simulink model "APB_Model0_v03_Test"  (R2020b)
settings: Solver=ode45  StartTime=0.0  StopTime=inf  RelTol=1e-3
undefined symbols (not defined in the file or in its folder): calb_Driver_acce, calb_Driver_bttn, calb_Driver_EmrBrk, calb_Driver_Prss, G_Fclamp, G_Kmot, G_Rmot, G_Stroke, G_SwOmega, GEN3, PbcDataStorageRequest_t
libraries: etargetslib x26, Lib_Op_Hndl x4, simulink x2, PbcOut_Checksum x2
(part 1 of 5)
settings Model: DataDictionary=APB_ModelDic.sldd  Creator=ISA1DRY  LastModifiedBy=OMO1DRY
settings SolverCC: ZeroCrossControl=DisableAll  ZeroCrossAlgorithm=Adaptive
settings DebuggingCC: IgnoredZcDiagnostic=none

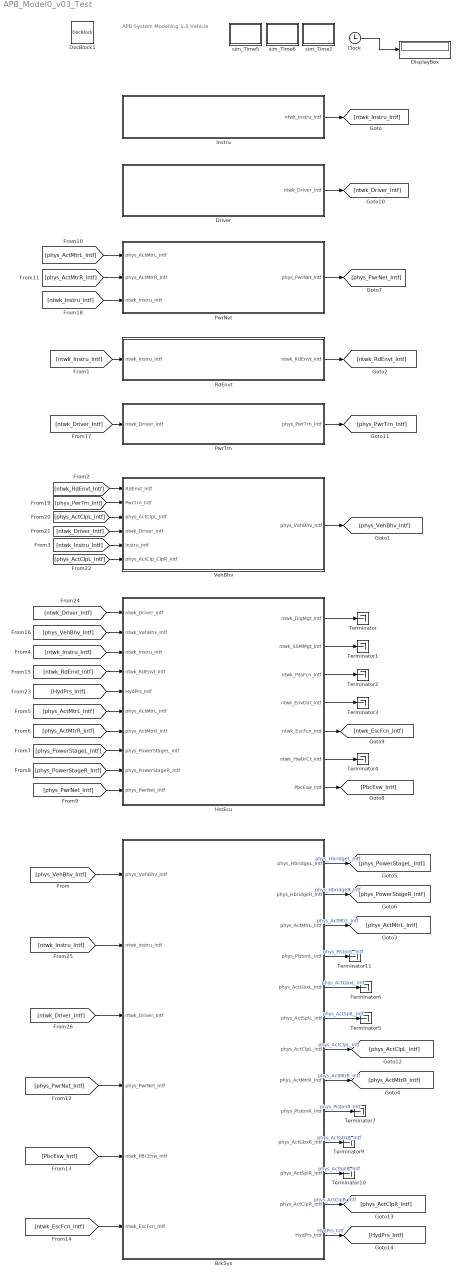
== system APB_Model0_v03_Test ==
  note: APB System Modelling
      | 1.0 Vehicle
  BrkSys : Subsystem
  Clock : Clock
  DisplayBox : Display
  DocBlock1 : simulink/Model-Wide Utilities/DocBlock  DocumentType=Text
      content=|
      | TyDate = 5 May 2023
      | Updated by = ALI ISSA
      | Model name = APB System Modeling
      | level = 02
      | version = 03
      |
      | Description
      |
      | New APB Model with the improved architecture...
  Driver : Subsystem
  HstEcu : Subsystem
  Instru : Subsystem
  PwrNet : Subsystem
  PwrTrn : Subsystem
  RdEnvt : Subsystem
  Terminator{,1..7,9..11} (11 alike) : Terminator
  VehBhv : Subsystem
  sim_Time1 : Subsystem
      mask Display: disp('Plot');
  sim_Time5 : Subsystem
      settings: OpenFcn=clear;
      mask Display: disp('clear');
  sim_Time6 : Subsystem
      settings: OpenFcn=|
      | startupNew_2;
      | Data_IntegDRYJPN3;
      mask Display: disp('load\nstartup');
  wires:
  Instru/1(ntwk_Instru_Intf) -> [ntwk_Instru_Intf]
  Driver/1(ntwk_Driver_Intf) -> [ntwk_Driver_Intf]
  [ntwk_Instru_Intf] -> RdEnvt/1(ntwk_Instru_Intf)
  [phys_ActMtrL_Intf] -> PwrNet/1(phys_ActMtrL_Intf)
  [phys_ActMtrR_Intf] -> PwrNet/2(phys_ActMtrR_Intf)
  [ntwk_Instru_Intf] -> PwrNet/3(ntwk_Instru_Intf)
  PwrNet/1(phys_PwrNet_Intf) -> [phys_PwrNet_Intf]
  RdEnvt/1(ntwk_RdEnvt_Intf) -> [ntwk_RdEnvt_Intf]
  [ntwk_Driver_Intf] -> PwrTrn/1(ntwk_Driver_Intf)
  PwrTrn/1(phys_PwrTrn_Intf) -> [phys_PwrTrn_Intf]
  [ntwk_RdEnvt_Intf] -> VehBhv/1(RdEnvt_Intf)
  VehBhv/1(phys_VehBhv_Intf) -> [phys_VehBhv_Intf]
  [phys_PwrTrn_Intf] -> VehBhv/2(PwrTrn_Intf)
  [phys_ActClpL_Intf] -> VehBhv/3(phys_ActClpL_Intf)
  [ntwk_Driver_Intf] -> VehBhv/4(ntwk_Driver_Intf)
  [ntwk_Instru_Intf] -> VehBhv/5(Instru_Intf)
  [phys_ActClpL_Intf] -> VehBhv/6(phys_ActClp_ClpR_Intf)
  [phys_PowerStageL_Intf] -> HstEcu/8(phys_PowerStageL_Intf)
  [phys_PowerStageR_Intf] -> HstEcu/9(phys_PowerStageR_Intf)
  [phys_PwrNet_Intf] -> HstEcu/10(phys_PwrNet_Intf)
  [phys_ActMtrL_Intf] -> HstEcu/6(phys_ActMtrL_Intf)
  [ntwk_Driver_Intf] -> HstEcu/1(ntwk_Driver_Intf)
  [phys_VehBhv_Intf] -> HstEcu/2(ntwk_VehBhv_Intf)
  [ntwk_Instru_Intf] -> HstEcu/3(ntwk_Instru_Intf)
  [ntwk_RdEnvt_Intf] -> HstEcu/4(ntwk_RdEnvt_Intf)
  [HydPrs_Intf] -> HstEcu/5(HydPrs_Intf)
  [phys_ActMtrR_Intf] -> HstEcu/7(phys_ActMtrR_Intf)
  HstEcu/7(PbcEsw_Intf) -> [PbcEsw_Intf]
  HstEcu/5(ntwk_EscFcn_Intf) -> [ntwk_EscFcn_Intf]
  HstEcu/1(ntwk_DigMgt_Intf) -> Terminator/1
  HstEcu/3(ntwk_PdsFcn_Intf) -> Terminator2/1
  HstEcu/2(ntwk_SSMMgt_Intf) -> Terminator1/1
  HstEcu/4(ntwk_EnvDat_Intf) -> Terminator3/1
  HstEcu/6(ntwk_HwDrCt_Intf) -> Terminator4/1
  [phys_PwrNet_Intf] -> BrkSys/4(phys_PwrNet_Intf)
  [PbcEsw_Intf] -> BrkSys/5(ntwk_PBCEsw_Intf)
  [ntwk_EscFcn_Intf] -> BrkSys/6(ntwk_EscFcn_Intf)
  [phys_VehBhv_Intf] -> BrkSys/1(phys_VehBhv_Intf)
  [ntwk_Instru_Intf] -> BrkSys/2(ntwk_Instru_Intf)
  [ntwk_Driver_Intf] -> BrkSys/3(ntwk_Driver_Intf)
  BrkSys/13(HydPrs_Intf) -> [HydPrs_Intf]  "HydPrs_Intf"
  BrkSys/1(phys_HbridgeL_Intf) -> [phys_PowerStageL_Intf]  "phys_HbridgeL_Intf"
  BrkSys/2(phys_HbridgeR_Intf) -> [phys_PowerStageR_Intf]  "phys_HbridgeR_Intf"
  BrkSys/3(phys_ActMtrL_Intf) -> [phys_ActMtrL_Intf]  "phys_ActMtrL_Intf"
  BrkSys/8(phys_ActMtrR_Intf) -> [phys_ActMtrR_Intf]  "phys_ActMtrR_Intf"
  BrkSys/5(phys_ActGbxL_Intf) -> Terminator6/1  "phys_ActGbxL_Intf"
  BrkSys/6(phys_ActSplL_Intf) -> Terminator5/1  "phys_ActSplL_Intf"
  BrkSys/7(phys_ActClpL_Intf) -> [phys_ActClpL_Intf]  "phys_ActClpL_Intf"
  BrkSys/11(phys_ActSplR_Intf) -> Terminator10/1  "phys_ActSplR_Intf"
  BrkSys/12(phys_ActClpR_Intf) -> [phys_ActClpR_Intf]  "phys_ActClpR_Intf"
  BrkSys/10(phys_ActGbxR_Intf) -> Terminator9/1  "phys_ActGbxR_Intf"
  BrkSys/4(phys_PistonL_Intf) -> Terminator11/1  "phys_PistonL_Intf"
  BrkSys/9(phys_PistonR_Intf) -> Terminator7/1  "phys_PistonR_Intf"
  Clock/1 -> DisplayBox/1

== system APB_Model0_v03_Test/BrkSys ==
  phys_VehBhv_Intf : Inport
  ntwk_Instru_Intf : Inport  Port=2
  ntwk_Driver_Intf : Inport  Port=3
  phys_PwrNet_Intf : Inport  Port=4
  ntwk_PBCEsw_Intf : Inport  Port=5
  ntwk_EscFcn_Intf : Inport  Port=6
  Subsystem Reference : Subsystem  ReferencedSubsystem=Ssys_BrkSysAPB_v02_0
  phys_HbridgeL_Intf : Outport
  phys_HbridgeR_Intf : Outport  Port=2
  phys_ActMtrL_Intf : Outport  Port=3
  phys_PistonL_Intf : Outport  Port=4
  phys_ActGbxL_Intf : Outport  Port=5
  phys_ActSplL_Intf : Outport  Port=6
  phys_ActClpL_Intf : Outport  Port=7
  phys_ActMtrR_Intf : Outport  Port=8
  phys_PistonR_Intf : Outport  Port=9
  phys_ActGbxR_Intf : Outport  Port=10
  phys_ActSplR_Intf : Outport  Port=11
  phys_ActClpR_Intf : Outport  Port=12
  HydPrs_Intf : Outport  Port=13
  wires:
  Subsystem Reference/9 -> phys_ActGbxR_Intf/1  "phys_ActGbxR_Intf"
  Subsystem Reference/4 -> phys_ActGbxL_Intf/1  "phys_ActGbxL_Intf"
  Subsystem Reference/12 -> phys_HbridgeR_Intf/1  "phys_HbridgeR_Intf"
  Subsystem Reference/13 -> HydPrs_Intf/1  "HydPrs_Intf"
  Subsystem Reference/8 -> phys_PistonR_Intf/1  "phys_PistonR_Intf"
  ntwk_EscFcn_Intf/1 -> Subsystem Reference/6
  Subsystem Reference/11 -> phys_ActClpR_Intf/1  "phys_ActClpR_Intf"
  Subsystem Reference/7 -> phys_ActMtrR_Intf/1  "phys_ActMtrR_Intf"
  Subsystem Reference/3 -> phys_PistonL_Intf/1  "phys_PistonL_Intf"
  Subsystem Reference/10 -> phys_ActSplR_Intf/1  "phys_ActSplR_Intf"
  phys_VehBhv_Intf/1 -> Subsystem Reference/1
  Subsystem Reference/6 -> phys_ActClpL_Intf/1  "phys_ActClpL_Intf"
  ntwk_Instru_Intf/1 -> Subsystem Reference/2
  ntwk_Driver_Intf/1 -> Subsystem Reference/3
  Subsystem Reference/5 -> phys_ActSplL_Intf/1  "phys_ActSplL_Intf"
  Subsystem Reference/1 -> phys_HbridgeL_Intf/1  "phys_HbridgeL_Intf"
  phys_PwrNet_Intf/1 -> Subsystem Reference/4
  ntwk_PBCEsw_Intf/1 -> Subsystem Reference/5
  Subsystem Reference/2 -> phys_ActMtrL_Intf/1  "phys_ActMtrL_Intf"

== system APB_Model0_v03_Test/Driver ==
  Cmpt_DriverAPB_v01_0_Test : Subsystem
  Subsystem1 : Subsystem
  ntwk_Driver_Intf : Outport
  wires:
  Cmpt_DriverAPB_v01_0_Test/1(calb_Driver_bttn) -> Subsystem1/1(calb_Driver_bttn)  "calb_Driver_bttn"
  Cmpt_DriverAPB_v01_0_Test/2(calb_Driver_Prss) -> Subsystem1/2(calb_Driver_Prss)  "calb_Driver_Prss"
  Cmpt_DriverAPB_v01_0_Test/4(calb_Driver_EmrBrk) -> Subsystem1/4(calb_Driver_EmrBrk)  "calb_Driver_EmrBrk"
  Subsystem1/1(ntwk_Driver_Intf) -> ntwk_Driver_Intf/1  "ntwk_Driver_Intf"
  Cmpt_DriverAPB_v01_0_Test/3(calb_Driver_acce) -> Subsystem1/3(calb_Driver_acce)  "calb_Driver_acce"

== system APB_Model0_v03_Test/HstEcu ==
  note: Scheduler
  ntwk_Driver_Intf : Inport
  ntwk_VehBhv_Intf : Inport  Port=2
  ntwk_Instru_Intf : Inport  Port=3
  ntwk_RdEnvt_Intf : Inport  Port=4
  HydPrs_Intf : Inport  Port=5
  phys_ActMtrL_Intf : Inport  Port=6
  phys_ActMtrR_Intf : Inport  Port=7
  phys_PowerStageL_Intf : Inport  Port=8
  phys_PowerStageR_Intf : Inport  Port=9
  phys_PwrNet_Intf : Inport  Port=10
  Chart1 : Stateflow chart  TreatAsAtomicUnit=on
  Function-Call Generator2 : simulink/Ports & Subsystems/Function-Call Generator  sample_time=0.001  numberOfIterations=1  DisallowWideOutput=off
  PBC : Subsystem
  Rate Transition{1..9,16} (10 alike) : RateTransition  Integrity=off  OutPortSampleTime=0.001
  Ssys_HstEcu0_v01 : Subsystem
  ntwk_DigMgt_Intf : Outport
  ntwk_SSMMgt_Intf : Outport  Port=2
  ntwk_PdsFcn_Intf : Outport  Port=3
  ntwk_EnvDat_Intf : Outport  Port=4
  ntwk_EscFcn_Intf : Outport  Port=5
  ntwk_HwDrCt_Intf : Outport  Port=6
  PbcEsw_Intf : Outport  Port=7
  wires:
  phys_ActMtrL_Intf/1 -> Rate Transition16/1
  phys_ActMtrR_Intf/1 -> Rate Transition1/1
  phys_PowerStageL_Intf/1 -> Rate Transition2/1
  phys_PowerStageR_Intf/1 -> Rate Transition3/1
  phys_PwrNet_Intf/1 -> Rate Transition4/1
  ntwk_Driver_Intf/1 -> Rate Transition5/1
  ntwk_VehBhv_Intf/1 -> Rate Transition6/1
  ntwk_Instru_Intf/1 -> Rate Transition7/1
  ntwk_RdEnvt_Intf/1 -> Rate Transition8/1
  HydPrs_Intf/1 -> Rate Transition9/1
  Ssys_HstEcu0_v01/2(ntwk_SSMMgt_Intf) -> PBC/3(ntwk_SSMMgt_Intf), ntwk_SSMMgt_Intf/1  "ntwk_SSMMgt_Intf"
  Ssys_HstEcu0_v01/3(ntwk_DigMgt_Intf) -> ntwk_DigMgt_Intf/1, PBC/4(ntwk_DigMgt_Intf)  "ntwk_DigMgt_Intf"
  Ssys_HstEcu0_v01/4(ntwk_EscFcn_Intf) -> ntwk_EscFcn_Intf/1, PBC/8(ntwk_EscFcn_Intf)  "ntwk_EscFcn_Intf"
  Ssys_HstEcu0_v01/5(ntwk_PdsFcn_Intf) -> PBC/5(ntwk_PdsFcn_Intf), ntwk_PdsFcn_Intf/1  "ntwk_PdsFcn_Intf"
  Ssys_HstEcu0_v01/6(ntwk_EnvDat_Intf) -> PBC/6(ntwk_EnvDat_Intf), ntwk_EnvDat_Intf/1  "ntwk_EnvDat_Intf"
  Ssys_HstEcu0_v01/1(ntwk_HwDrCt_Intf) -> ntwk_HwDrCt_Intf/1, PBC/7(ntwk_HwDrCt_Intf)  "ntwk_HwDrCt_Intf"
  Chart1/2(Init()) -> [Init]
  Function-Call Generator2/1 -> Chart1/Trigger
  Chart1/3(Step()) -> [Cyclic]
  Chart1/1(HostCall()) -> [HostCall]
  Rate Transition16/1 -> Ssys_HstEcu0_v01/1(phys_ActMtrL_Intf)
  Rate Transition1/1 -> Ssys_HstEcu0_v01/2(phys_ActMtrR_Intf)
  Rate Transition2/1 -> Ssys_HstEcu0_v01/3(phys_PowerStageL_Intf)
  Rate Transition3/1 -> Ssys_HstEcu0_v01/4(phys_PowerStageR_Intf)
  Rate Transition4/1 -> Ssys_HstEcu0_v01/5(phys_PwrNet_Intf)
  Rate Transition5/1 -> Ssys_HstEcu0_v01/6(ntwk_Driver_Intf)
  Rate Transition6/1 -> Ssys_HstEcu0_v01/7(ntwk_VehBhv_Intf)
  Rate Transition7/1 -> Ssys_HstEcu0_v01/9(ntwk_Instru_Intf)
  Rate Transition8/1 -> Ssys_HstEcu0_v01/10(ntwk_RdEnvt_Intf)
  Rate Transition9/1 -> Ssys_HstEcu0_v01/11(HydPrs_Intf)
  PBC/1(PbcEsw_Intf) -> Ssys_HstEcu0_v01/8(ntwk_PbcEsw_Intf), PbcEsw_Intf/1
  [HostCall] -> Ssys_HstEcu0_v01/12(Host_Callall)
  [Init] -> PBC/1(Init)
  [Cyclic] -> PBC/2(cyclic)

== system APB_Model0_v03_Test/Instru ==
  Cmpt_InstruAPB_v01_0 : Subsystem  ReferencedSubsystem=Cmpt_InstruAPB_v01_0
  Subsystem1 : Subsystem
  ntwk_Instru_Intf : Outport
  wires:
  Cmpt_InstruAPB_v01_0/38 -> Subsystem1/38(Instru_I_Mot_ESP_1)
  Cmpt_InstruAPB_v01_0/27 -> Subsystem1/27(Instru_MotorVoltageSensorR)
  Cmpt_InstruAPB_v01_0/3 -> Subsystem1/3(Instru_DriverStateTestSignalL)
  Cmpt_InstruAPB_v01_0/37 -> Subsystem1/37(Instru_I_Valves)
  Cmpt_InstruAPB_v01_0/17 -> Subsystem1/17(Instru_WhlPulsTestSignalRR)
  Cmpt_InstruAPB_v01_0/15 -> Subsystem1/15(Instru_WhlPulsTestSignalFR)
  Cmpt_InstruAPB_v01_0/11 -> Subsystem1/11(Instru_WhlSpdTestSignalRR)
  Cmpt_InstruAPB_v01_0/7 -> Subsystem1/7(Instru_WhlPrsReliabTestSignalFR)
  Subsystem1/1(ntwk_Instru_Intf) -> ntwk_Instru_Intf/1  "ntwk_Instru_Intf"
  Cmpt_InstruAPB_v01_0/36 -> Subsystem1/36(Instru_DriVolTestSignal)
  Cmpt_InstruAPB_v01_0/16 -> Subsystem1/16(Instru_WhlPulsTestSignalRL)
  Cmpt_InstruAPB_v01_0/20 -> Subsystem1/20(Instru_WhlPrsTestSignalFL)
  Cmpt_InstruAPB_v01_0/4 -> Subsystem1/4(Instru_DriverStateTestSignalR)
  Cmpt_InstruAPB_v01_0/9 -> Subsystem1/9(Instru_WhlPrsReliabTestSignalRR)
  Cmpt_InstruAPB_v01_0/10 -> Subsystem1/10(Instru_WhlSpdTestSignalRL)
  Cmpt_InstruAPB_v01_0/6 -> Subsystem1/6(Instru_WhlPrsReliabTestSignalFL)
  Cmpt_InstruAPB_v01_0/2 -> Subsystem1/2(Instru_FrontWhSpSns)
  Cmpt_InstruAPB_v01_0/19 -> Subsystem1/19(Instru_WhlPrsTestSignalRR)
  Cmpt_InstruAPB_v01_0/8 -> Subsystem1/8(Instru_WhlPrsReliabTestSignalRL)
  Cmpt_InstruAPB_v01_0/23 -> Subsystem1/23(Instru_FreeTravelR)
  Cmpt_InstruAPB_v01_0/22 -> Subsystem1/22(Instru_FreeTravelL)
  Cmpt_InstruAPB_v01_0/1 -> Subsystem1/1(Instru_RearWhSpSns)
  Cmpt_InstruAPB_v01_0/18 -> Subsystem1/18(Instru_WhlPrsTestSignalRL)
  Cmpt_InstruAPB_v01_0/5 -> Subsystem1/5(Instru_SlpTestSignal)
  Cmpt_InstruAPB_v01_0/32 -> Subsystem1/32(Instru_InitState)
  Cmpt_InstruAPB_v01_0/12 -> Subsystem1/12(Instru_WhlSpdTestSignalFL)
  Cmpt_InstruAPB_v01_0/33 -> Subsystem1/33(Instru_HpsDelay)
  Cmpt_InstruAPB_v01_0/30 -> Subsystem1/30(Instru_InitForceL)
  Cmpt_InstruAPB_v01_0/31 -> Subsystem1/31(Instru_InitForceR)
  Cmpt_InstruAPB_v01_0/26 -> Subsystem1/26(Instru_MotorVoltageSensorL)
  Cmpt_InstruAPB_v01_0/34 -> Subsystem1/34(Instru_HpsAckDelay)
  Cmpt_InstruAPB_v01_0/21 -> Subsystem1/21(Instru_WhlPrsTestSignalFR)
  Cmpt_InstruAPB_v01_0/35 -> Subsystem1/35(Instru_ReqDefault)
  Cmpt_InstruAPB_v01_0/28 -> Subsystem1/28(Instru_ActMGU_effL)
  Cmpt_InstruAPB_v01_0/29 -> Subsystem1/29(Instru_ActMGU_effR)
  Cmpt_InstruAPB_v01_0/24 -> Subsystem1/24(Instru_MotorCurrentSensorL)
  Cmpt_InstruAPB_v01_0/25 -> Subsystem1/25(Instru_MotorCurrentSensorR)
  Cmpt_InstruAPB_v01_0/13 -> Subsystem1/13(Instru_WhlSpdTestSignalFR)
  Cmpt_InstruAPB_v01_0/14 -> Subsystem1/14(Instru_WhlPulsTestSignalFL)

== system APB_Model0_v03_Test/PwrNet ==
  phys_ActMtrL_Intf : Inport
  phys_ActMtrR_Intf : Inport  Port=2
  ntwk_Instru_Intf : Inport  Port=3
  Cmpt_PwrNetAPB_v03_0_ : Subsystem  ReferencedSubsystem=Cmpt_PwrNetAPB_v03_0
  Subsystem1 : Subsystem
  Subsystem9 : Subsystem
  phys_PwrNet_Intf : Outport
  wires:
  Cmpt_PwrNetAPB_v03_0_/1 -> Subsystem1/1(phys_PwrNet_VOut_L)
  Cmpt_PwrNetAPB_v03_0_/2 -> Subsystem1/2(phys_PwrNet_VOut_R)
  Subsystem1/1(phys_PwrNet_Intf) -> phys_PwrNet_Intf/1
  Subsystem9/1(Out1) -> Cmpt_PwrNetAPB_v03_0_/1
  Subsystem9/2(phys_ActMtr_Current_R) -> Cmpt_PwrNetAPB_v03_0_/2
  Subsystem9/3(Instru_I_Valves) -> Cmpt_PwrNetAPB_v03_0_/3
  Subsystem9/4(Instru_I_Mot_ESP_1) -> Cmpt_PwrNetAPB_v03_0_/4
  phys_ActMtrL_Intf/1 -> Subsystem9/1(phys_ActMtr_Intf)
  phys_ActMtrR_Intf/1 -> Subsystem9/2(phys_ActMtrR_Intf)
  ntwk_Instru_Intf/1 -> Subsystem9/3(Instru_Int)
  Cmpt_PwrNetAPB_v03_0_/3 -> Subsystem1/3(phys_PwrNet_VIn)

== system APB_Model0_v03_Test/PwrTrn ==
  ntwk_Driver_Intf : Inport
  Cmpt_PwrTrnAPB_v01_0 : Subsystem  ReferencedSubsystem=Cmpt_PwrTrnAPB_v01_0
  Subsystem1 : Subsystem
  Subsystem2 : Subsystem
  phys_PwrTrn_Intf : Outport  VectorParamsAs1DForOutWhenUnconnected=off
  wires:
  ntwk_Driver_Intf/1 -> Subsystem2/1(ntwk_Driver_Intf)
  Subsystem2/1(phys_PwrTrn_Torq) -> Cmpt_PwrTrnAPB_v01_0/1
  Cmpt_PwrTrnAPB_v01_0/1 -> Subsystem1/1(In1)
  Subsystem1/1(phys_PwrTrn_Intf) -> phys_PwrTrn_Intf/1  "phys_PwrTrn_Intf"

== system APB_Model0_v03_Test/RdEnvt ==
  ntwk_Instru_Intf : Inport
  Cmpt_RdEnvtAPB_v01_0 : Subsystem  ReferencedSubsystem=Cmpt_RdEnvtAPB_v01_0
  Subsystem1 : Subsystem
  Subsystem2 : Subsystem
  ntwk_RdEnvt_Intf : Outport
  wires:
  Cmpt_RdEnvtAPB_v01_0/3 -> Subsystem1/3(In3)  "phys_RdEnvt_Slope"
  ntwk_Instru_Intf/1 -> Subsystem2/1(ntwk_Instru_Intf)
  Subsystem2/1(Out1) -> Cmpt_RdEnvtAPB_v01_0/1
  Subsystem1/1(ntwk_RdEnvt_Intf) -> ntwk_RdEnvt_Intf/1
  Cmpt_RdEnvtAPB_v01_0/2 -> Subsystem1/2(In2)  "phys_RdEnvt_Fslop"
  Cmpt_RdEnvtAPB_v01_0/1 -> Subsystem1/1(In1)  "phys_RdEnvt_LgAc"

== system APB_Model0_v03_Test/VehBhv ==
  RdEnvt_Intf : Inport
  PwrTrn_Intf : Inport  Port=2
  phys_ActClpL_Intf : Inport  Port=3
  ntwk_Driver_Intf : Inport  Port=4
  Instru_Intf : Inport  Port=5
  phys_ActClp_ClpR_Intf : Inport  Port=6
  Ssys_VehBhvAPB_v01_0 : Subsystem  ReferencedSubsystem=Ssys_VehBhvAPB_v01_0
  Subsystem : Subsystem
  phys_VehBhv_Intf : Outport
  wires:
  phys_ActClp_ClpR_Intf/1 -> Ssys_VehBhvAPB_v01_0/6
  PwrTrn_Intf/1 -> Ssys_VehBhvAPB_v01_0/2
  Subsystem/1(phys_VehBhv_Intf) -> phys_VehBhv_Intf/1
  Instru_Intf/1 -> Ssys_VehBhvAPB_v01_0/5
  RdEnvt_Intf/1 -> Ssys_VehBhvAPB_v01_0/1
  Ssys_VehBhvAPB_v01_0/2 -> Subsystem/2(In2)
  Ssys_VehBhvAPB_v01_0/1 -> Subsystem/1(In1)
  ntwk_Driver_Intf/1 -> Ssys_VehBhvAPB_v01_0/4
  phys_ActClpL_Intf/1 -> Ssys_VehBhvAPB_v01_0/3

== system APB_Model0_v03_Test/sim_Time1 ==

== system APB_Model0_v03_Test/sim_Time5 ==

== system APB_Model0_v03_Test/sim_Time6 ==

== system APB_Model0_v03_Test/Driver/Cmpt_DriverAPB_v01_0_Test ==
  Constant : Constant  Value=calb_Driver_bttn
  Constant1 : Constant  Value=calb_Driver_Prss
  Constant2 : Constant  Value=calb_Driver_acce
  Constant3 : Constant  Value=calb_Driver_EmrBrk
  From Workspace : FromWorkspace  Commented=on  VariableName=Button_state  SampleTime=-1
  From Workspace1 : FromWorkspace  Commented=on  VariableName=couplemoteur
  From Workspace2 : FromWorkspace  Commented=on  VariableName=a_Pressin  SampleTime=-1
  Rate Transition : RateTransition
  Rate Transition1 : RateTransition
  Terminator : Terminator
  calb_Driver_bttn : Outport
  calb_Driver_Prss : Outport  Port=2
  calb_Driver_acce : Outport  Port=3
  calb_Driver_EmrBrk : Outport  Port=4
  wires:
  Constant3/1 -> calb_Driver_EmrBrk/1  "calb_Driver_EmrBrk"
  Constant1/1 -> Rate Transition/1  "calb_Driver_Prss"
  Rate Transition/1 -> calb_Driver_Prss/1
  Rate Transition1/1 -> calb_Driver_bttn/1
  From Workspace2/1 -> Terminator/1  "calb_Driver_Prss"
  Constant/1 -> Rate Transition1/1  "calb_Driver_bttn"
  Constant2/1 -> calb_Driver_acce/1  "calb_Driver_acce"

== system APB_Model0_v03_Test/Driver/Subsystem1 ==
  calb_Driver_bttn : Inport
  calb_Driver_Prss : Inport  Port=2
  calb_Driver_acce : Inport  Port=3
  calb_Driver_EmrBrk : Inport  Port=4
  Bus Creator : BusCreator  Inputs=4
  ntwk_Driver_Intf : Outport
  wires:
  calb_Driver_EmrBrk/1 -> Bus Creator/4
  calb_Driver_acce/1 -> Bus Creator/3
  calb_Driver_bttn/1 -> Bus Creator/1
  Bus Creator/1 -> ntwk_Driver_Intf/1
  calb_Driver_Prss/1 -> Bus Creator/2

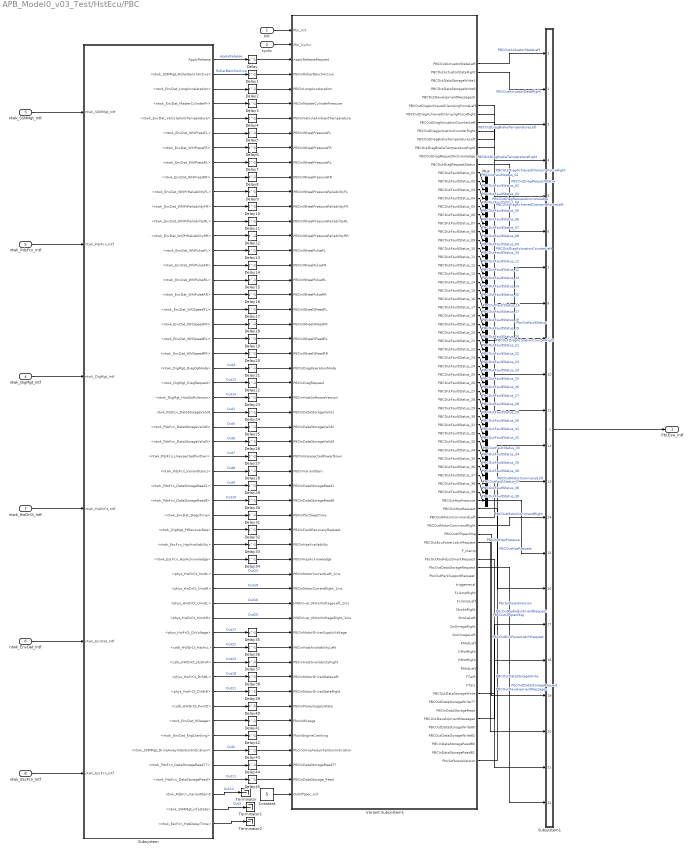
== system APB_Model0_v03_Test/HstEcu/PBC ==
  Init : Inport
  cyclic : Inport  Port=2
  ntwk_SSMMgt_Intf : Inport  Port=3
  ntwk_DigMgt_Intf : Inport  Port=4
  ntwk_PdsFcn_Intf : Inport  Port=5
  ntwk_EnvDat_Intf : Inport  Port=6
  ntwk_HwDrCt_Intf : Inport  Port=7
  ntwk_EscFcn_Intf : Inport  Port=8
  Constant : Constant  Value=5
  Delay{,1,9..12,21..22,24..27,32..34,38..43} (21 alike) : Delay  DelayLength=1  InitialCondition=5  SampleTime=0.01
  Delay{2..8,13..20,23,28..31,35,44..45} (23 alike) : Delay  DelayLength=1  SampleTime=0.01
  Delay36 : Delay  DelayLength=1  InitialCondition=54  SampleTime=0.01
  Delay37 : Delay  DelayLength=1  InitialCondition=54  SampleTime=0.01
  Mux : Mux  Inputs=39
  Subsystem : Subsystem
  Subsystem1 : Subsystem
  Terminator : Terminator
  Terminator1 : Terminator
  Terminator2 : Terminator
  Variant Subsystem1 : Subsystem  Variant=on
  PbcEsw_Intf : Outport
  wires:
  ntwk_SSMMgt_Intf/1 -> Subsystem/1(ntwk_SSMMgt_Intf)
  ntwk_PdsFcn_Intf/1 -> Subsystem/2(ntwk_PdsFcn_Intf)
  ntwk_DigMgt_Intf/1 -> Subsystem/3(ntwk_DigMgt_Intf)
  ntwk_HwDrCt_Intf/1 -> Subsystem/4(ntwk_HwDrCt_Intf)
  ntwk_EnvDat_Intf/1 -> Subsystem/5(ntwk_EnvDat_Intf)
  ntwk_EscFcn_Intf/1 -> Subsystem/6(ntwk_EscFcn_Intf)
  Subsystem/1(ApplyRelease) -> Delay/1  "ApplyRelease"
  Subsystem/2(<ntwk_SSMMgt_RollerBenchActive>) -> Delay1/1  "RollerBenchActive"
  Subsystem/3(<ntwk_EnvDat_LongAcceleration>) -> Delay2/1
  Subsystem/4(<ntwk_EnvDat_MasterCylinderPr>) -> Delay3/1
  Subsystem/5(<ntwk_EnvDat_VehicleAmbTemperature>) -> Delay4/1
  Subsystem/6(<ntwk_EnvDat_WhlPressFL>) -> Delay5/1
  Subsystem/7(<ntwk_EnvDat_WhlPressFR>) -> Delay6/1
  Subsystem/8(<ntwk_EnvDat_WhlPressRL>) -> Delay7/1
  Subsystem/9(<ntwk_EnvDat_WhlPressRR>) -> Delay8/1
  Subsystem/10(<ntwk_EnvDat_WhlPrReliabilityFL>) -> Delay9/1
  Subsystem/11(<ntwk_EnvDat_WhlPrReliabilityFR>) -> Delay10/1
  Subsystem/12(<ntwk_EnvDat_WhlPrReliabilityRL>) -> Delay11/1
  Subsystem/13(<ntwk_EnvDat_WhlPrReliabilityRR>) -> Delay12/1
  Subsystem/14(<ntwk_EnvDat_WhlPulseFL>) -> Delay13/1
  Subsystem/15(<ntwk_EnvDat_WhlPulseFR>) -> Delay14/1
  Subsystem/16(<ntwk_EnvDat_WhlPulseRL>) -> Delay15/1
  Subsystem/17(<ntwk_EnvDat_WhlPulseRR>) -> Delay16/1
  Subsystem/18(<ntwk_EnvDat_WhlSpeedFL>) -> Delay17/1
  Subsystem/19(<ntwk_EnvDat_WhlSpeedFR>) -> Delay18/1
  Subsystem/20(<ntwk_EnvDat_WhlSpeedRL>) -> Delay19/1
  Subsystem/21(<ntwk_EnvDat_WhlSpeedRR>) -> Delay20/1
  Subsystem/22(<ntwk_DigMgt_DiagOpMode>) -> Delay21/1  "Out4"
  Subsystem/23(<ntwk_DigMgt_DiagRequest>) -> Delay22/1  "Out13"
  Subsystem/24(<ntwk_DigMgt_HostSoftVersion>) -> Delay23/1  "Out14"
  Subsystem/25(ntwk_PdsFcn_DataStorageValid1) -> Delay24/1  "Out1"
  Subsystem/26(<ntwk_PdsFcn_DataStorageValid2>) -> Delay25/1  "Out5"
  Subsystem/27(<ntwk_PdsFcn_DataStorageValid3>) -> Delay26/1  "Out6"
  Subsystem/28(<ntwk_PdsFcn_UnexpectedPwrDwn>) -> Delay27/1  "Out7"
  Subsystem/29(<ntwk_PdsFcn_VariantItem1>) -> Delay28/1  "Out8"
  Subsystem/30(<ntwk_PdsFcn_DataStorageRead1>) -> Delay29/1  "Out9"
  Subsystem/31(<ntwk_PdsFcn_DataStorageRead9>) -> Delay30/1  "Out10"
  Subsystem/33(<ntwk_DigMgt_FtRecoverReq>) -> Delay32/1
  Subsystem/34(<ntwk_EscFcn_HpsAvailability>) -> Delay33/1
  Subsystem/35(<ntwk_EscFcn_HpsAcknowledge>) -> Delay34/1
  Subsystem/36(<phys_HwDrCt_ImotL>) -> Variant Subsystem1/38(PBCInMotorCurrentLeft_1ms)  "Out15"
  Subsystem/37(<phys_HwDrCt_ImotR>) -> Variant Subsystem1/39(PBCInMotorCurrentRight_1ms)  "Out19"
  Subsystem/32(<ntwk_EnvDat_SleepTime>) -> Delay31/1
  Subsystem/38(<phys_HwDrCt_UmotL>) -> Variant Subsystem1/40(HWDriver_MotorVoltageLeft_1ms)  "Out16"
  Subsystem/39(<phys_HwDrCt_UmotR>) -> Variant Subsystem1/41(HWDriver_MotorVoltageRight_1ms)  "Out20"
  Subsystem/40(<phys_HwFrCt_DrVoltage>) -> Delay35/1  "Out17"
  Subsystem/41(<calb_HWDrCt_HstAvL>) -> Delay36/1  "Out22"
  Subsystem/42(<calb_HWDrCt_HstAvR>) -> Delay37/1  "Out23"
  Subsystem/43(<phys_HwFrCt_DrSttL>) -> Delay38/1  "Out18"
  Subsystem/44(<phys_HwFrCt_DrSttR>) -> Delay39/1  "Out21"
  Subsystem/45(<calb_HWDrCt_Pwrstt>) -> Delay40/1
  Subsystem/46(<ntwk_EnvDat_Mileage>) -> Delay41/1
  Subsystem/47(<ntwk_EnvDat_EngCranking>) -> Delay42/1
  Subsystem/48(<ntwk_SSMMgt_DriveAwayIntentionIndication>) -> Delay43/1  "Out2"
  Subsystem/49(<ntwk_PdsFcn_DataStorageRead77>) -> Delay44/1
  Subsystem/50(<ntwk_PdsFcn_DataStorageRead>) -> Delay45/1  "Out11"
  Subsystem/51(ntwk_PdsFcn_VariantItem0) -> Terminator/1  "Out12"
  Subsystem/52(<ntwk_SSMMgt_infostate>) -> Terminator1/1  "Out3"
  Subsystem/53(<ntwk_EscFcn_HpsDelayTime>) -> Terminator2/1
  Variant Subsystem1/84(PbcSoftwareVersion) -> Subsystem1/12(PbcSoftwareVersion)  "PbcSoftwareVersion"
  Variant Subsystem1/1(PBCOutActuatorStateLeft) -> Subsystem1/1(PBCOutActuatorStateLeft)  "PBCOutActuatorStateLeft"
  Variant Subsystem1/2(PBCOutActuatorStateRight) -> Subsystem1/2(PBCOutActuatorStateRight)  "PBCOutActuatorStateRight"
  Variant Subsystem1/55(PBCOutMotorCommandLeft) -> Subsystem1/13(In1)  "PBCOutMotorCommandLeft"
  Variant Subsystem1/56(PBCOutMotorCommandRight) -> Subsystem1/14(In2)  "PBCOutMotorCommandRight"
  Variant Subsystem1/10(PBCOutDiagBrakeTemperatureLeft) -> Subsystem1/3(In3)  "PBCOutDiagBrakeTemperatureLeft"
  Variant Subsystem1/11(PBCOutDiagBrakeTemperatureRight) -> Subsystem1/4(In4)  "PBCOutDiagBrakeTemperatureRight"
  Variant Subsystem1/12(PBCOutDiagRequestAcknowledge) -> Subsystem1/5(In5)  "PBCOutDiagRequestAcknowledge"
  Variant Subsystem1/13(PBCOutDiagRequestStatus) -> Subsystem1/6(In6)  "PBCOutDiagRequestStatus"
  Variant Subsystem1/14(PBCOutFaultStatus_01) -> Mux/1  "PBCOutFaultStatus_01"
  Variant Subsystem1/15(PBCOutFaultStatus_02) -> Mux/2  "PBCOutFaultStatus_02"
  Variant Subsystem1/16(PBCOutFaultStatus_03) -> Mux/3  "PBCOutFaultStatus_03"
  Variant Subsystem1/17(PBCOutFaultStatus_04) -> Mux/4  "PBCOutFaultStatus_04"
  Variant Subsystem1/18(PBCOutFaultStatus_05) -> Mux/5  "PBCOutFaultStatus_05"
  Variant Subsystem1/19(PBCOutFaultStatus_06) -> Mux/6  "PBCOutFaultStatus_06"
  Variant Subsystem1/20(PBCOutFaultStatus_07) -> Mux/7  "PBCOutFaultStatus_07"
  Variant Subsystem1/21(PBCOutFaultStatus_08) -> Mux/8  "PBCOutFaultStatus_08"
  Variant Subsystem1/22(PBCOutFaultStatus_09) -> Mux/9  "PBCOutFaultStatus_09"
  Variant Subsystem1/23(PBCOutFaultStatus_10) -> Mux/10  "PBCOutFaultStatus_10"
  Variant Subsystem1/24(PBCOutFaultStatus_11) -> Mux/11  "PBCOutFaultStatus_11"
  Variant Subsystem1/25(PBCOutFaultStatus_12) -> Mux/12  "PBCOutFaultStatus_12"
  Variant Subsystem1/26(PBCOutFaultStatus_13) -> Mux/13  "PBCOutFaultStatus_13"
  Variant Subsystem1/27(PBCOutFaultStatus_14) -> Mux/14  "PBCOutFaultStatus_14"
  Variant Subsystem1/28(PBCOutFaultStatus_15) -> Mux/15  "PBCOutFaultStatus_15"
  Variant Subsystem1/29(PBCOutFaultStatus_16) -> Mux/16  "PBCOutFaultStatus_16"
  Variant Subsystem1/30(PBCOutFaultStatus_17) -> Mux/17  "PBCOutFaultStatus_17"
  Variant Subsystem1/31(PBCOutFaultStatus_18) -> Mux/18  "PBCOutFaultStatus_18"
  Variant Subsystem1/32(PBCOutFaultStatus_19) -> Mux/19  "PBCOutFaultStatus_19"
  Variant Subsystem1/33(PBCOutFaultStatus_20) -> Mux/20  "PBCOutFaultStatus_20"
  Variant Subsystem1/34(PBCOutFaultStatus_21) -> Mux/21  "PBCOutFaultStatus_21"
  Variant Subsystem1/35(PBCOutFaultStatus_22) -> Mux/22  "PBCOutFaultStatus_22"
  Variant Subsystem1/36(PBCOutFaultStatus_23) -> Mux/23  "PBCOutFaultStatus_23"
  Variant Subsystem1/37(PBCOutFaultStatus_24) -> Mux/24  "PBCOutFaultStatus_24"
  Variant Subsystem1/38(PBCOutFaultStatus_25) -> Mux/25  "PBCOutFaultStatus_25"
  Variant Subsystem1/39(PBCOutFaultStatus_26) -> Mux/26  "PBCOutFaultStatus_26"
  Variant Subsystem1/40(PBCOutFaultStatus_27) -> Mux/27  "PBCOutFaultStatus_27"
  Variant Subsystem1/41(PBCOutFaultStatus_28) -> Mux/28  "PBCOutFaultStatus_28"
  Variant Subsystem1/42(PBCOutFaultStatus_29) -> Mux/29  "PBCOutFaultStatus_29"
  Variant Subsystem1/43(PBCOutFaultStatus_30) -> Mux/30  "PBCOutFaultStatus_30"
  Variant Subsystem1/44(PBCOutFaultStatus_31) -> Mux/31  "PBCOutFaultStatus_31"
  Variant Subsystem1/45(PBCOutFaultStatus_32) -> Mux/32  "PBCOutFaultStatus_32"
  Variant Subsystem1/46(PBCOutFaultStatus_33) -> Mux/33  "PBCOutFaultStatus_33"
  Variant Subsystem1/47(PBCOutFaultStatus_34) -> Mux/34  "PBCOutFaultStatus_34"
  Variant Subsystem1/48(PBCOutFaultStatus_35) -> Mux/35  "PBCOutFaultStatus_35"
  Variant Subsystem1/49(PBCOutFaultStatus_36) -> Mux/36  "PBCOutFaultStatus_36"
  Variant Subsystem1/50(PBCOutFaultStatus_37) -> Mux/37  "PBCOutFaultStatus_37"
  Variant Subsystem1/51(PBCOutFaultStatus_38) -> Mux/38  "PBCOutFaultStatus_38"
  Variant Subsystem1/52(PBCOutFaultStatus_39) -> Mux/39  "PBCOutFaultStatus_39"
  Mux/1 -> Subsystem1/7(In7)  "PbcOutfaultStatus"
  Variant Subsystem1/6(PBCOutDiagAchievedClampingForceLeft) -> Subsystem1/8(In8)  "PBCOutDiagAchievedClampingForceLeft"
  Variant Subsystem1/7(PBCOutDiagAchievedClampingForceRight) -> Subsystem1/9(In9)  "PBCOutDiagAchievedClampingForceRight"
  Variant Subsystem1/8(PBCOutDiagActuationCounterLeft) -> Subsystem1/10(In10)  "PBCOutDiagActuationCounterLeft"
  Variant Subsystem1/9(PBCOutDiagActuationCounterRight) -> Subsystem1/11(In11)  "PBCOutDiagActuationCounterRight"
  Variant Subsystem1/53(PBCOutHpsPressure) -> Subsystem1/15(In12)  "PBCOutHpsPressure"
  Variant Subsystem1/54(PBCOutHpsRequest) -> Subsystem1/16(In13)  "PBCOutHpsRequest"
  Variant Subsystem1/76(PBCOutDataStorageWrite) -> Subsystem1/17(In14)  "PBCOutDataStorageWrite"
  Variant Subsystem1/79(PBCOutDevelopmentMessages) -> Subsystem1/18(In15)  "PBCOutDevelopmentMessages"
  Variant Subsystem1/57(PBCOutOfSpecMsg) -> Subsystem1/19(In16)  "PBCOutOfSpecMsg"
  Variant Subsystem1/58(PBCOutEcuPowerLatchRequest) -> Subsystem1/20(In17)  "PBCOutEcuPowerLatchRequest"
  Variant Subsystem1/60(PbcOutPadAdjustmentRequest) -> Subsystem1/21(In18)  "PbcOutPadAdjustmentRequest"
  Variant Subsystem1/61(PbcOutDataStorageRequest) -> Subsystem1/22(In19)  "PbcOutDataStorageRequest"
  Subsystem1/1(PbcEsw_Intf) -> PbcEsw_Intf/1
  Init/1 -> Variant Subsystem1/1(Pbc_Init)
  cyclic/1 -> Variant Subsystem1/2(Pbc_Cyclic)
  Constant/1 -> Variant Subsystem1/53(OutOfSpec_Init)
  Delay/1 -> Variant Subsystem1/3(ApplyReleaseRequest)
  Delay2/1 -> Variant Subsystem1/5(PBCInLongAcceleration)
  Delay3/1 -> Variant Subsystem1/6(PBCInMasterCylinderPressure)
  Delay4/1 -> Variant Subsystem1/7(PBCInVehicleAmbientTemperature)
  Delay5/1 -> Variant Subsystem1/8(PBCInWheelPressureFL)
  Delay6/1 -> Variant Subsystem1/9(PBCInWheelPressureFR)
  Delay7/1 -> Variant Subsystem1/10(PBCInWheelPressureRL)
  Delay8/1 -> Variant Subsystem1/11(PBCInWheelPressureRR)
  Delay9/1 -> Variant Subsystem1/12(PBCInWheelPressureReliabilityFL)
  Delay10/1 -> Variant Subsystem1/13(PBCInWheelPressureReliabilityFR)
  Delay11/1 -> Variant Subsystem1/14(PBCInWheelPressureReliabilityRL)
  Delay12/1 -> Variant Subsystem1/15(PBCInWheelPressureReliabilityRR)
  Delay13/1 -> Variant Subsystem1/16(PBCInWheelPulseFL)
  Delay14/1 -> Variant Subsystem1/17(PBCInWheelPulseFR)
  Delay15/1 -> Variant Subsystem1/18(PBCInWheelPulseRL)
  Delay16/1 -> Variant Subsystem1/19(PBCInWheelPulseRR)
  Delay17/1 -> Variant Subsystem1/20(PBCInWheelSPeedFL)
  Delay18/1 -> Variant Subsystem1/21(PBCInWheelSPeedFR)
  Delay19/1 -> Variant Subsystem1/22(PBCInWheelSPeedRL)
  Delay20/1 -> Variant Subsystem1/23(PBCInWheelSPeedRR)
  Delay21/1 -> Variant Subsystem1/24(PBCInDiagOperationMode)
  Delay22/1 -> Variant Subsystem1/25(PBCInDiagRequest)
  Delay23/1 -> Variant Subsystem1/26(PBCinHostSoftwareVersion)
  Delay24/1 -> Variant Subsystem1/27(PBCInDataStorageValid1)
  Delay25/1 -> Variant Subsystem1/28(PBCInDataStorageValid2)
  Delay26/1 -> Variant Subsystem1/29(PBCInDataStorageValid3)
  Delay27/1 -> Variant Subsystem1/30(PBCInUnexpectedPowerDown)
  Delay28/1 -> Variant Subsystem1/31(PBCInVariantItem)
  Delay29/1 -> Variant Subsystem1/32(PBCInDataStorageRead1)
  Delay30/1 -> Variant Subsystem1/33(PBCInDataStorageRead9)
  Delay31/1 -> Variant Subsystem1/34(PBCInPbcSleepTime)
  Delay32/1 -> Variant Subsystem1/35(PBCInFaultRecoveryRequest)
  Delay33/1 -> Variant Subsystem1/36(PBCInHpsAvailability)
  Delay34/1 -> Variant Subsystem1/37(PBCInHpsAcknowledge)
  Delay35/1 -> Variant Subsystem1/42(PBCInMotorDriverSupplyVoltage)
  Delay36/1 -> Variant Subsystem1/43(PBCinHostAvailabilityLeft)
  Delay37/1 -> Variant Subsystem1/44(PBCinHostAvailabilityRight)
  Delay38/1 -> Variant Subsystem1/45(PBCInMotorDriverStateLeft)
  Delay39/1 -> Variant Subsystem1/46(PBCInMotorDriverStateRight)
  Delay40/1 -> Variant Subsystem1/47(PBCInPowerSupplyState)
  Delay41/1 -> Variant Subsystem1/48(PbcInMileage)
  Delay42/1 -> Variant Subsystem1/49(PbcInEngineCranking)
  Delay44/1 -> Variant Subsystem1/51(PBCInDataStorageRead77)
  Delay45/1 -> Variant Subsystem1/52(PBCInDataStorage_Read)
  Delay43/1 -> Variant Subsystem1/50(PbcInDriveAwayIntentionIndication)
  Delay1/1 -> Variant Subsystem1/4(PBCInRollerBenchActive)

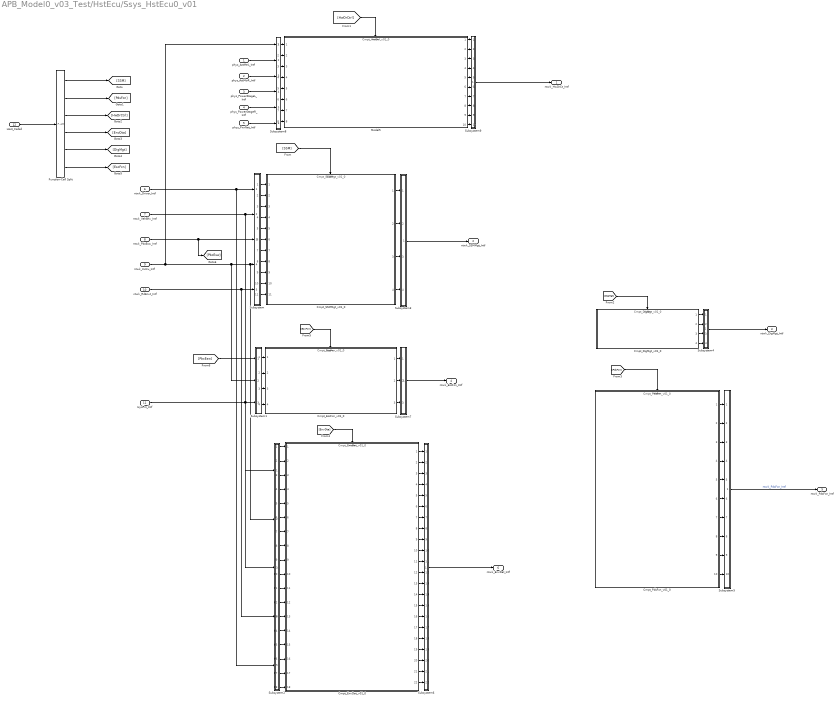
== system APB_Model0_v03_Test/HstEcu/Ssys_HstEcu0_v01 ==
  phys_ActMtrL_Intf : Inport
  phys_ActMtrR_Intf : Inport  Port=2
  phys_PowerStageL_Intf : Inport  Port=3
  phys_PowerStageR_Intf : Inport  Port=4
  phys_PwrNet_Intf : Inport  Port=5
  ntwk_Driver_Intf : Inport  Port=6
  ntwk_VehBhv_Intf : Inport  Port=7
  ntwk_PbcEsw_Intf : Inport  Port=8  LockScale=on
  ntwk_Instru_Intf : Inport  Port=9
  ntwk_RdEnvt_Intf : Inport  Port=10
  HydPrs_Intf : Inport  Port=11
  Host_Callall : Inport  Port=12
  Cmpt_DigMgt_v01_0 : ModelReference  ModelNameDialog=Cmpt_DigMgt_v01_0.slx  SimulationMode=Normal  ModelReferenceVersion=1.11  TriggerPortName=Host_Call  TriggerPortTriggerType=function-call  TriggerPortStatesWhenEnabling=held
  Cmpt_EnvDat_v01_0 : ModelReference  ModelNameDialog=Cmpt_EnvDat_v01_0.slx  SimulationMode=Normal  ModelReferenceVersion=1.33  TriggerPortName=Host_Call  TriggerPortTriggerType=function-call  TriggerPortStatesWhenEnabling=held
  Cmpt_EscFcn_v01_0 : ModelReference  ModelNameDialog=Cmpt_EscFcn_v01_0.slx  SimulationMode=Normal  ModelReferenceVersion=1.12  TriggerPortName=Host_Call  TriggerPortTriggerType=function-call  TriggerPortStatesWhenEnabling=held
  Cmpt_PdsFcn_v01_0 : ModelReference  ModelNameDialog=Cmpt_PdsFcn_v01_0.slx  SimulationMode=Normal  ModelReferenceVersion=1.10  TriggerPortName=Host_Call  TriggerPortTriggerType=function-call  TriggerPortStatesWhenEnabling=held
  Cmpt_SSMMgt_v01_0 : ModelReference  ModelNameDialog=Cmpt_SSMMgt_v01_0.slx  SimulationMode=Normal  ModelReferenceVersion=1.34  TriggerPortName=Host_Call  TriggerPortTriggerType=function-call  TriggerPortStatesWhenEnabling=held
  Function-Call Split : FunctionCallSplit  IconShape=distinctive  NumOutputPorts=6  OutputPortLayout=default
  Model5 : ModelReference  ModelNameDialog=Cmpt_HwCtrl_v01_0.slx  SimulationMode=Normal  ModelReferenceVersion=1.15  TriggerPortName=Host_Call  TriggerPortTriggerType=function-call  TriggerPortStatesWhenEnabling=held
  Subsystem : Subsystem
  Subsystem1 : Subsystem
  Subsystem2 : Subsystem
  Subsystem3 : Subsystem
  Subsystem4 : Subsystem
  Subsystem5 : Subsystem
  Subsystem6 : Subsystem
  Subsystem7 : Subsystem
  Subsystem8 : Subsystem
  Subsystem9 : Subsystem
  ntwk_HwDrCt_Intf : Outport
  ntwk_SSMMgt_Intf : Outport  Port=2
  ntwk_DigMgt_Intf : Outport  Port=3
  ntwk_EscFcn_Intf : Outport  Port=4
  ntwk_PdsFcn_Intf : Outport  Port=5
  ntwk_EnvDat_Intf : Outport  Port=6
  wires:
  Cmpt_EnvDat_v01_0/14 -> Subsystem6/14(In14)
  Cmpt_PdsFcn_v01_0/6 -> Subsystem5/6(In6)
  Subsystem1/1(ntwk_PbcEsw_HpsReq) -> Cmpt_EscFcn_v01_0/1
  Subsystem8/8(Out7) -> Model5/8
  phys_PowerStageL_Intf/1 -> Subsystem8/4(phys_PowerStageL_Intf)
  ntwk_RdEnvt_Intf/1 -> Subsystem/5(ntwk_RdEnvt_Intf), Subsystem2/4(ntwk_RdEnvt_Intf)
  Cmpt_DigMgt_v01_0/3 -> Subsystem4/3(In3)
  phys_PowerStageR_Intf/1 -> Subsystem8/5(phys_PowerStageR_Intf)
  Subsystem8/1(Out1) -> Model5/1
  Cmpt_EnvDat_v01_0/8 -> Subsystem6/8(In8)
  Subsystem2/18(Out2) -> Cmpt_EnvDat_v01_0/18
  Subsystem8/2(Out2) -> Model5/2
  Subsystem/8(Out7) -> Cmpt_SSMMgt_v01_0/8
  ntwk_Instru_Intf/1 -> Subsystem/4(ntwk_Instru_Intf), Subsystem2/2(ntwk_Instru_Intf), Subsystem1/2(ntwk_Instru_Intf), Subsystem8/1(ntwk_Instru_Intf)
  phys_ActMtrR_Intf/1 -> Subsystem8/3(phys_ActMtrR_Intf)
  Subsystem2/9(Out9) -> Cmpt_EnvDat_v01_0/9
  Subsystem2/17(Out17) -> Cmpt_EnvDat_v01_0/17
  phys_ActMtrL_Intf/1 -> Subsystem8/2(phys_ActMtrL_Intf)
  ntwk_Driver_Intf/1 -> Subsystem/1(ntwk_Driver_Intf), Subsystem2/5(ntwk_Driver_Intf)
  ntwk_VehBhv_Intf/1 -> Subsystem/2(ntwk_VehBhv_Intf), Subsystem2/3(ntwk_VehBhv_Intf)
  Subsystem/7(Out6) -> Cmpt_SSMMgt_v01_0/7
  Cmpt_PdsFcn_v01_0/5 -> Subsystem5/5(In5)
  Cmpt_EnvDat_v01_0/2 -> Subsystem6/2(In2)
  Subsystem8/4(Out4) -> Model5/4
  Cmpt_SSMMgt_v01_0/3 -> Subsystem3/3(ntwk_SSMMgt_infostate)
  Cmpt_EnvDat_v01_0/13 -> Subsystem6/13(In13)
  Subsystem1/3(Out1) -> Cmpt_EscFcn_v01_0/3
  Subsystem8/6(Out8) -> Model5/6
  Subsystem/2(ntwk_PbcEsw_ActSttL) -> Cmpt_SSMMgt_v01_0/2
  Cmpt_DigMgt_v01_0/2 -> Subsystem4/2(ntwk_DigMgt_DiagRequest)
  Subsystem/5(Out1) -> Cmpt_SSMMgt_v01_0/5
  Subsystem8/5(Out5) -> Model5/5
  Subsystem8/3(Out3) -> Model5/3
  ntwk_PbcEsw_Intf/1 -> [PbcEsw], Subsystem/3(ntwk_PbcEsw_Intf)
  Subsystem2/6(Out6) -> Cmpt_EnvDat_v01_0/6
  Subsystem8/7(Out6) -> Model5/7
  Subsystem6/1(ntwk_EnvDat_Intf) -> ntwk_EnvDat_Intf/1
  Subsystem/3(ntwk_PbcEsw_ActSttR) -> Cmpt_SSMMgt_v01_0/3
  Cmpt_EnvDat_v01_0/5 -> Subsystem6/5(In5)
  Subsystem2/11(Out11) -> Cmpt_EnvDat_v01_0/11
  Cmpt_PdsFcn_v01_0/3 -> Subsystem5/3(In3)
  Cmpt_EnvDat_v01_0/1 -> Subsystem6/1(In1)
  Cmpt_EnvDat_v01_0/6 -> Subsystem6/6(In6)
  Cmpt_EnvDat_v01_0/4 -> Subsystem6/4(In4)
  Subsystem/4(ntwk_PbcEsw_PadAdjReq) -> Cmpt_SSMMgt_v01_0/4
  Cmpt_PdsFcn_v01_0/8 -> Subsystem5/8(In8)
  Subsystem5/1(ntwk_PdsFcn_Intf) -> ntwk_PdsFcn_Intf/1  "ntwk_PdsFcn_Intf"
  Subsystem/9(Out4) -> Cmpt_SSMMgt_v01_0/9
  Subsystem2/16(Out16) -> Cmpt_EnvDat_v01_0/16
  Subsystem/6(Out8) -> Cmpt_SSMMgt_v01_0/6
  Cmpt_EnvDat_v01_0/3 -> Subsystem6/3(In3)
  Subsystem2/2(Out1) -> Cmpt_EnvDat_v01_0/2
  Cmpt_PdsFcn_v01_0/2 -> Subsystem5/2(In2)
  Cmpt_EscFcn_v01_0/2 -> Subsystem7/2(In2)
  Subsystem4/1(ntwk_DigMgt_Intf) -> ntwk_DigMgt_Intf/1
  Subsystem2/10(Out10) -> Cmpt_EnvDat_v01_0/10
  Cmpt_EscFcn_v01_0/1 -> Subsystem7/1(In1)
  Subsystem1/4(ntwk_PbcEsw_HpsPressOut) -> Cmpt_EscFcn_v01_0/4
  Cmpt_EnvDat_v01_0/21 -> Subsystem6/21(In21)
  Cmpt_PdsFcn_v01_0/1 -> Subsystem5/1(In1)
  Cmpt_EnvDat_v01_0/11 -> Subsystem6/11(In11)
  Subsystem2/7(Out7) -> Cmpt_EnvDat_v01_0/7
  Cmpt_EnvDat_v01_0/7 -> Subsystem6/7(In7)
  Cmpt_EnvDat_v01_0/19 -> Subsystem6/19(In19)
  Cmpt_EnvDat_v01_0/15 -> Subsystem6/15(In15)
  Subsystem2/5(Out5) -> Cmpt_EnvDat_v01_0/5
  Subsystem/1(Out2) -> Cmpt_SSMMgt_v01_0/1
  Subsystem7/1(ntwk_EscFcn_Intf) -> ntwk_EscFcn_Intf/1
  Cmpt_EnvDat_v01_0/9 -> Subsystem6/9(In9)
  Subsystem/10(Out3) -> Cmpt_SSMMgt_v01_0/10
  Cmpt_EnvDat_v01_0/18 -> Subsystem6/18(In18)
  Cmpt_PdsFcn_v01_0/9 -> Subsystem5/9(In9)
  Cmpt_PdsFcn_v01_0/4 -> Subsystem5/4(In4)
  Cmpt_EnvDat_v01_0/12 -> Subsystem6/12(In12)
  Subsystem2/15(Out15) -> Cmpt_EnvDat_v01_0/15
  Cmpt_SSMMgt_v01_0/1 -> Subsystem3/1(ntwk_SSMMgt_ApplyRelRequest)
  Subsystem2/13(Out13) -> Cmpt_EnvDat_v01_0/13
  Subsystem3/1(ntwk_SSMMgt_Intf) -> ntwk_SSMMgt_Intf/1
  Cmpt_EnvDat_v01_0/16 -> Subsystem6/16(In16)
  Cmpt_SSMMgt_v01_0/4 -> Subsystem3/4(ntwk_SSMMgt_RollerBenchActive)
  Cmpt_EnvDat_v01_0/17 -> Subsystem6/17(In17)
  Cmpt_EnvDat_v01_0/22 -> Subsystem6/22(In22)
  Subsystem9/1(ntwk_HwDrCt_Intf) -> ntwk_HwDrCt_Intf/1
  Subsystem2/12(Out12) -> Cmpt_EnvDat_v01_0/12
  Cmpt_SSMMgt_v01_0/2 -> Subsystem3/2(ntwk_SSMMgt_DriveAwayIntentionIndication)
  Cmpt_DigMgt_v01_0/1 -> Subsystem4/1(ntwk_DigMgt_DiagOpMode)
  Subsystem/11(Out5) -> Cmpt_SSMMgt_v01_0/11
  Cmpt_EscFcn_v01_0/3 -> Subsystem7/3(In3)
  Cmpt_EnvDat_v01_0/10 -> Subsystem6/10(In10)
  Cmpt_EnvDat_v01_0/20 -> Subsystem6/20(In20)
  Cmpt_PdsFcn_v01_0/7 -> Subsystem5/7(In7)
  Subsystem2/8(Out8) -> Cmpt_EnvDat_v01_0/8
  Subsystem2/14(Out14) -> Cmpt_EnvDat_v01_0/14
  HydPrs_Intf/1 -> Subsystem1/3(HydPrs_Intf), Subsystem2/1(HydPrs_Intf)
  Subsystem1/2(Out2) -> Cmpt_EscFcn_v01_0/2
  Subsystem2/1(X) -> Cmpt_EnvDat_v01_0/1
  Subsystem2/4(Out4) -> Cmpt_EnvDat_v01_0/4
  Subsystem2/3(Out3) -> Cmpt_EnvDat_v01_0/3
  phys_PwrNet_Intf/1 -> Subsystem8/6(phys_PwrNet_Intf)
  Model5/1 -> Subsystem9/1(In1)
  Model5/2 -> Subsystem9/2(In2)
  Model5/3 -> Subsystem9/3(In3)
  Model5/4 -> Subsystem9/4(In4)
  Model5/5 -> Subsystem9/5(In5)
  Model5/6 -> Subsystem9/6(In6)
  Model5/7 -> Subsystem9/7(In7)
  Model5/8 -> Subsystem9/8(In8)
  Model5/9 -> Subsystem9/9(In9)
  Model5/10 -> Subsystem9/10(In10)
  Cmpt_DigMgt_v01_0/4 -> Subsystem4/4(In1)
  Cmpt_PdsFcn_v01_0/10 -> Subsystem5/10(In10)
  Host_Callall/1 -> Function-Call Split/1
  Function-Call Split/1 -> [SSM]
  Function-Call Split/2 -> [PdsFcn]
  [SSM] -> Cmpt_SSMMgt_v01_0/Trigger
  Function-Call Split/3 -> [HwDrCtrl]
  Function-Call Split/4 -> [EnvDta]
  Function-Call Split/5 -> [DigMgt]
  Function-Call Split/6 -> [EscFcn]
  [HwDrCtrl] -> Model5/Trigger
  [DigMgt] -> Cmpt_DigMgt_v01_0/Trigger
  [PdsFcn] -> Cmpt_PdsFcn_v01_0/Trigger
  [EnvDta] -> Cmpt_EnvDat_v01_0/Trigger
  [EscFcn] -> Cmpt_EscFcn_v01_0/Trigger
  [PbcEsw] -> Subsystem1/1(ntwk_PbcEsw_Intf)

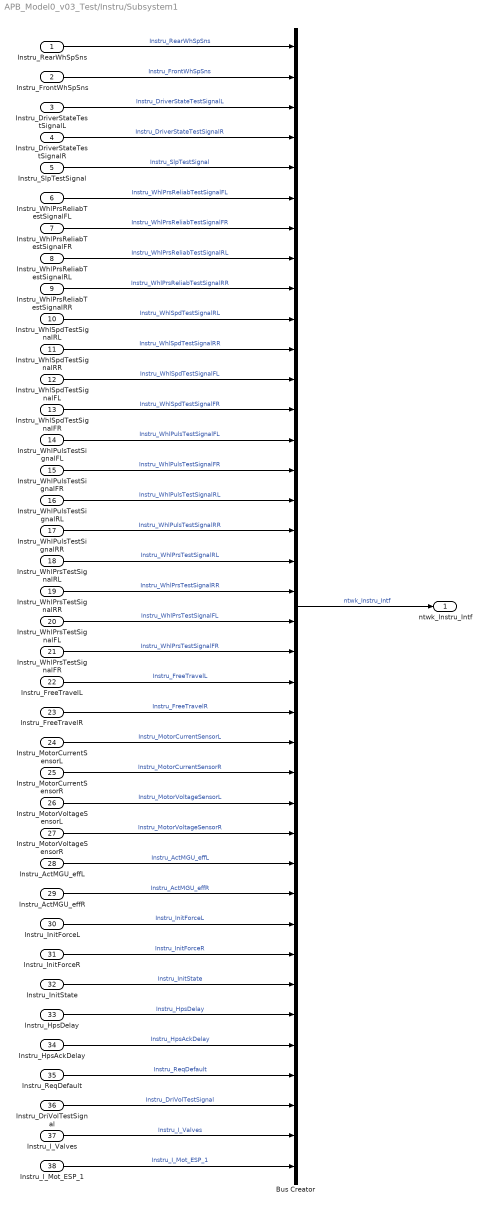
== system APB_Model0_v03_Test/Instru/Subsystem1 ==
  Instru_RearWhSpSns : Inport
  Instru_FrontWhSpSns : Inport  Port=2
  Instru_DriverStateTestSignalL : Inport  Port=3
  Instru_DriverStateTestSignalR : Inport  Port=4
  Instru_SlpTestSignal : Inport  Port=5
  Instru_WhlPrsReliabTestSignalFL : Inport  Port=6
  Instru_WhlPrsReliabTestSignalFR : Inport  Port=7
  Instru_WhlPrsReliabTestSignalRL : Inport  Port=8
  Instru_WhlPrsReliabTestSignalRR : Inport  Port=9
  Instru_WhlSpdTestSignalRL : Inport  Port=10
  Instru_WhlSpdTestSignalRR : Inport  Port=11
  Instru_WhlSpdTestSignalFL : Inport  Port=12
  Instru_WhlSpdTestSignalFR : Inport  Port=13
  Instru_WhlPulsTestSignalFL : Inport  Port=14
  Instru_WhlPulsTestSignalFR : Inport  Port=15
  Instru_WhlPulsTestSignalRL : Inport  Port=16
  Instru_WhlPulsTestSignalRR : Inport  Port=17
  Instru_WhlPrsTestSignalRL : Inport  Port=18
  Instru_WhlPrsTestSignalRR : Inport  Port=19
  Instru_WhlPrsTestSignalFL : Inport  Port=20
  Instru_WhlPrsTestSignalFR : Inport  Port=21
  Instru_FreeTravelL : Inport  Port=22
  Instru_FreeTravelR : Inport  Port=23
  Instru_MotorCurrentSensorL : Inport  Port=24
  Instru_MotorCurrentSensorR : Inport  Port=25
  Instru_MotorVoltageSensorL : Inport  Port=26
  Instru_MotorVoltageSensorR : Inport  Port=27
  Instru_ActMGU_effL : Inport  Port=28
  Instru_ActMGU_effR : Inport  Port=29
  Instru_InitForceL : Inport  Port=30
  Instru_InitForceR : Inport  Port=31
  Instru_InitState : Inport  Port=32
  Instru_HpsDelay : Inport  Port=33
  Instru_HpsAckDelay : Inport  Port=34
  Instru_ReqDefault : Inport  Port=35
  Instru_DriVolTestSignal : Inport  Port=36
  Instru_I_Valves : Inport  Port=37
  Instru_I_Mot_ESP_1 : Inport  Port=38
  Bus Creator : BusCreator  Inputs=38
  ntwk_Instru_Intf : Outport
  wires:
  Bus Creator/1 -> ntwk_Instru_Intf/1  "ntwk_Instru_Intf"
  Instru_WhlSpdTestSignalFR/1 -> Bus Creator/13  "Instru_WhlSpdTestSignalFR"
  Instru_WhlSpdTestSignalFL/1 -> Bus Creator/12  "Instru_WhlSpdTestSignalFL"
  Instru_WhlSpdTestSignalRL/1 -> Bus Creator/10  "Instru_WhlSpdTestSignalRL"
  Instru_WhlSpdTestSignalRR/1 -> Bus Creator/11  "Instru_WhlSpdTestSignalRR"
  Instru_WhlPrsReliabTestSignalRR/1 -> Bus Creator/9  "Instru_WhlPrsReliabTestSignalRR"
  Instru_WhlPrsReliabTestSignalRL/1 -> Bus Creator/8  "Instru_WhlPrsReliabTestSignalRL"
  Instru_WhlPrsReliabTestSignalFR/1 -> Bus Creator/7  "Instru_WhlPrsReliabTestSignalFR"
  Instru_WhlPrsReliabTestSignalFL/1 -> Bus Creator/6  "Instru_WhlPrsReliabTestSignalFL"
  Instru_SlpTestSignal/1 -> Bus Creator/5  "Instru_SlpTestSignal"
  Instru_DriverStateTestSignalR/1 -> Bus Creator/4  "Instru_DriverStateTestSignalR"
  Instru_DriverStateTestSignalL/1 -> Bus Creator/3  "Instru_DriverStateTestSignalL"
  Instru_FrontWhSpSns/1 -> Bus Creator/2  "Instru_FrontWhSpSns"
  Instru_RearWhSpSns/1 -> Bus Creator/1  "Instru_RearWhSpSns"
  Instru_WhlPulsTestSignalFL/1 -> Bus Creator/14  "Instru_WhlPulsTestSignalFL"
  Instru_WhlPulsTestSignalFR/1 -> Bus Creator/15  "Instru_WhlPulsTestSignalFR"
  Instru_WhlPulsTestSignalRL/1 -> Bus Creator/16  "Instru_WhlPulsTestSignalRL"
  Instru_WhlPulsTestSignalRR/1 -> Bus Creator/17  "Instru_WhlPulsTestSignalRR"
  Instru_WhlPrsTestSignalRL/1 -> Bus Creator/18  "Instru_WhlPrsTestSignalRL"
  Instru_WhlPrsTestSignalRR/1 -> Bus Creator/19  "Instru_WhlPrsTestSignalRR"
  Instru_WhlPrsTestSignalFL/1 -> Bus Creator/20  "Instru_WhlPrsTestSignalFL"
  Instru_WhlPrsTestSignalFR/1 -> Bus Creator/21  "Instru_WhlPrsTestSignalFR"
  Instru_FreeTravelL/1 -> Bus Creator/22  "Instru_FreeTravelL"
  Instru_FreeTravelR/1 -> Bus Creator/23  "Instru_FreeTravelR"
  Instru_MotorCurrentSensorL/1 -> Bus Creator/24  "Instru_MotorCurrentSensorL"
  Instru_MotorCurrentSensorR/1 -> Bus Creator/25  "Instru_MotorCurrentSensorR"
  Instru_MotorVoltageSensorL/1 -> Bus Creator/26  "Instru_MotorVoltageSensorL"
  Instru_MotorVoltageSensorR/1 -> Bus Creator/27  "Instru_MotorVoltageSensorR"
  Instru_ActMGU_effL/1 -> Bus Creator/28  "Instru_ActMGU_effL"
  Instru_ActMGU_effR/1 -> Bus Creator/29  "Instru_ActMGU_effR"
  Instru_InitForceL/1 -> Bus Creator/30  "Instru_InitForceL"
  Instru_InitForceR/1 -> Bus Creator/31  "Instru_InitForceR"
  Instru_InitState/1 -> Bus Creator/32  "Instru_InitState"
  Instru_HpsDelay/1 -> Bus Creator/33  "Instru_HpsDelay"
  Instru_HpsAckDelay/1 -> Bus Creator/34  "Instru_HpsAckDelay"
  Instru_ReqDefault/1 -> Bus Creator/35  "Instru_ReqDefault"
  Instru_DriVolTestSignal/1 -> Bus Creator/36  "Instru_DriVolTestSignal"
  Instru_I_Valves/1 -> Bus Creator/37  "Instru_I_Valves"
  Instru_I_Mot_ESP_1/1 -> Bus Creator/38  "Instru_I_Mot_ESP_1"

== system APB_Model0_v03_Test/PwrNet/Subsystem1 ==
  phys_PwrNet_VOut_L : Inport
  phys_PwrNet_VOut_R : Inport  Port=2
  phys_PwrNet_VIn : Inport  Port=3
  Bus Creator : BusCreator  Inputs=3
  To Workspace : ToWorkspace  VariableName=phys_PwrNet_VIn  SaveFormat=Timeseries  SampleTime=0.01
  phys_PwrNet_Intf : Outport
  wires:
  Bus Creator/1 -> phys_PwrNet_Intf/1  "phys_PwrNet_Intf"
  phys_PwrNet_VOut_R/1 -> Bus Creator/2  "phys_PwrNet_VOut_R"
  phys_PwrNet_VOut_L/1 -> Bus Creator/1  "phys_PwrNet_VOut_L"
  phys_PwrNet_VIn/1 -> To Workspace/1, Bus Creator/3  "phys_PwrNet_VIn"

== system APB_Model0_v03_Test/PwrNet/Subsystem9 ==
  phys_ActMtr_Intf : Inport
  phys_ActMtrR_Intf : Inport  Port=2
  Instru_Int : Inport  Port=3
  Bus Selector : BusSelector  OutputSignals=phys_ActMtr_Current
  Bus Selector1 : BusSelector  OutputSignals=phys_ActMtr_Current
  Bus Selector2 : BusSelector  OutputSignals=Instru_I_Valves,Instru_I_Mot_ESP_1
  Out1 : Outport
  phys_ActMtr_Current_R : Outport  Port=2
  Instru_I_Valves : Outport  Port=3
  Instru_I_Mot_ESP_1 : Outport  Port=4
  wires:
  phys_ActMtr_Intf/1 -> Bus Selector/1
  phys_ActMtrR_Intf/1 -> Bus Selector1/1
  Bus Selector/1 -> Out1/1  "<phys_ActMtr_Current>"
  Bus Selector1/1 -> phys_ActMtr_Current_R/1  "<phys_ActMtr_Current>"
  Instru_Int/1 -> Bus Selector2/1
  Bus Selector2/1 -> Instru_I_Valves/1  "<Instru_I_Valves>"
  Bus Selector2/2 -> Instru_I_Mot_ESP_1/1  "<Instru_I_Mot_ESP_1>"

== system APB_Model0_v03_Test/PwrTrn/Subsystem1 ==
  In1 : Inport
  Bus Creator : BusCreator  Inputs=1
  phys_PwrTrn_Intf : Outport
  wires:
  In1/1 -> Bus Creator/1
  Bus Creator/1 -> phys_PwrTrn_Intf/1

== system APB_Model0_v03_Test/PwrTrn/Subsystem2 ==
  ntwk_Driver_Intf : Inport
  Bus Selector : BusSelector  OutputSignals=calb_Driver_acce
  phys_PwrTrn_Torq : Outport
  wires:
  ntwk_Driver_Intf/1 -> Bus Selector/1
  Bus Selector/1 -> phys_PwrTrn_Torq/1  "<calb_Driver_acce>"

== system APB_Model0_v03_Test/RdEnvt/Subsystem1 ==
  In1 : Inport
  In2 : Inport  Port=2
  In3 : Inport  Port=3
  Bus Creator : BusCreator  Inputs=3
  ntwk_RdEnvt_Intf : Outport
  wires:
  Bus Creator/1 -> ntwk_RdEnvt_Intf/1
  In2/1 -> Bus Creator/2
  In1/1 -> Bus Creator/1
  In3/1 -> Bus Creator/3

== system APB_Model0_v03_Test/RdEnvt/Subsystem2 ==
  ntwk_Instru_Intf : Inport
  Bus Selector : BusSelector  OutputSignals=Instru_SlpTestSignal
  Out1 : Outport
  wires:
  ntwk_Instru_Intf/1 -> Bus Selector/1
  Bus Selector/1 -> Out1/1  "<Instru_SlpTestSignal>"

== system APB_Model0_v03_Test/VehBhv/Subsystem ==
  In1 : Inport
  In2 : Inport  Port=2
  Bus Creator : BusCreator  Inputs=2
  phys_VehBhv_Intf : Outport
  wires:
  Bus Creator/1 -> phys_VehBhv_Intf/1  "phys_VehBhv_Intf"
  In1/1 -> Bus Creator/1
  In2/1 -> Bus Creator/2
